simulink model "LecturerFullAM"  (R2023a)
settings: Solver=FixedStepDiscrete  StartTime=0.0  StopTime=1  RelTol=1e-3
settings Model: Creator=Pedro  LastModifiedBy=Pedro

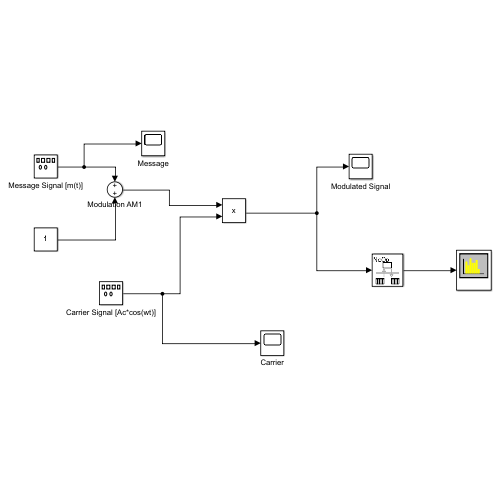
[thumbnail: Simulink's stored preview of the top-level diagram]
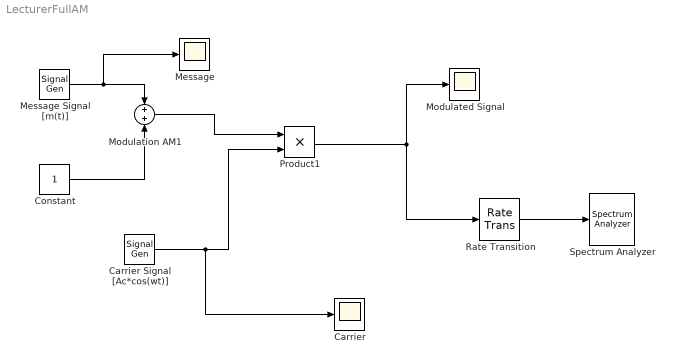
== system LecturerFullAM ==
  Carrier : Scope
  Carrier Signal [Ac*cos(wt)] : SignalGenerator  Frequency=100
  Constant : Constant
  Message : Scope
  Message Signal [m(t)] : SignalGenerator  Amplitude=0.5  Frequency=10
  Modulated Signal : Scope
  Modulation AM1 : Sum
  Product1 : Product
  Rate Transition : RateTransition  OutPortSampleTime=0.001
  Spectrum Analyzer : SpectrumAnalyzer  WindowPosition=[10.000000,108.000000,709.000000,500.000000,]  ScopeFrameLocation=window  SampleRateSource=Property  SampleRate=44.1e3  PlotAsTwoSidedSpectrum=off  FrequencyScale=Log  FrequencySpan=Start and stop frequencies  StartFrequency=20  StopFrequency=20e3  YLimits=[-1,1]  ColorLimits=[-20 80]  SelectedToolstripTab=spectrumAnalyzerToolstrip.spectralMaskTab  DefaultConfigurationName=spbscopes.SpectrumAnalyzerBlockCfg  IsFrequencyInputMode=0  FrequencyVectorPort=0  FrequencyVectorFromPort=0  FrequencyInputRBWPort=0  FrequencyInputRBWFromPort=0
  wires:
  Product1/1 -> Rate Transition/1, Modulated Signal/1
  Message Signal [m(t)]/1 -> Message/1, Modulation AM1/1
  Constant/1 -> Modulation AM1/2
  Modulation AM1/1 -> Product1/1
  Carrier Signal [Ac*cos(wt)]/1 -> Carrier/1, Product1/2
  Rate Transition/1 -> Spectrum Analyzer/1
